simulink model "Test_model"  (R2022a)
settings: Solver=FixedStepAuto  StartTime=0.0  StopTime=.01  FixedStep=1e-6  RelTol=1e-3
libraries: spsSeriesRLCBranchLib x3, spsVoltageMeasurementLib x2, spsControlledVoltageSourceLib x1, simulink x1, spspowerguiLib x1
settings Model: Creator=ducks  LastModifiedBy=ducks

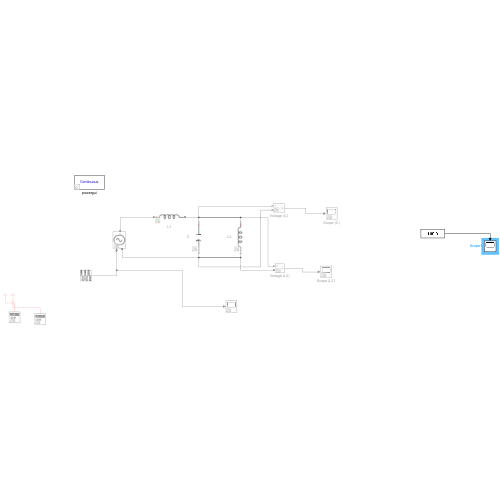
[thumbnail: Simulink's stored preview of the top-level diagram]
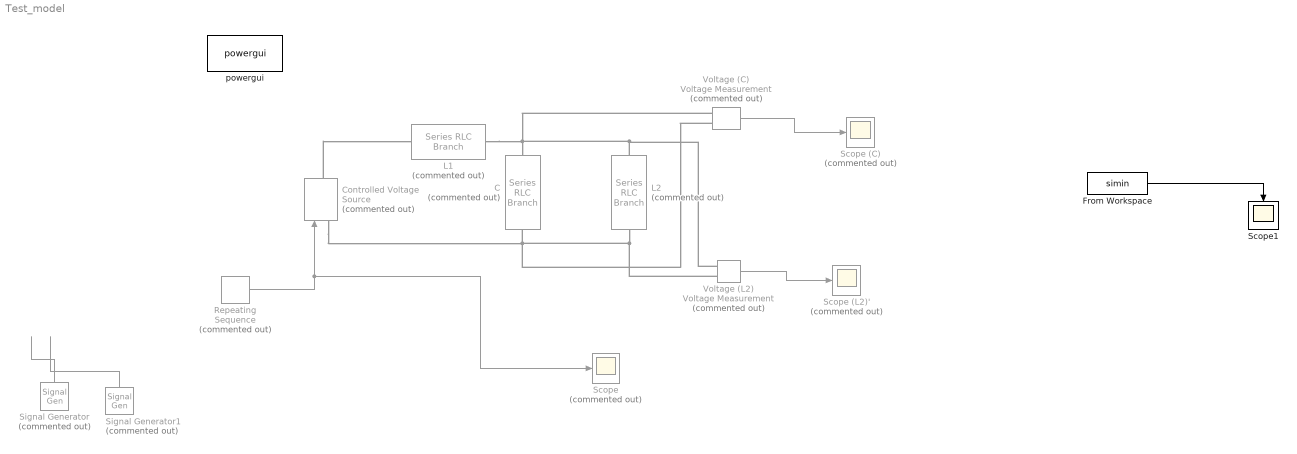
== system Test_model ==
  C : spsSeriesRLCBranchLib/Series RLC Branch  Commented=on  LConnTagsString=__new0  RConnTagsString=__new0  BranchType=C  Resistance=1  Inductance=1e-3  SetiL0=off  InitialCurrent=0  Capacitance=96e-6  Setx0=off  InitialVoltage=0  Measurements=None
  Controlled Voltage Source : spsControlledVoltageSourceLib/Controlled Voltage Source  Commented=on  Initialize=on  Source_Type=AC  Amplitude=0  Phase=0  Frequency=0  Measurements=None
  From Workspace : FromWorkspace  VariableName=simin
  L1 : spsSeriesRLCBranchLib/Series RLC Branch  Commented=on  LConnTagsString=__new0  RConnTagsString=__new0  BranchType=L  Resistance=1  Inductance=10e-6  SetiL0=off  InitialCurrent=0  Capacitance=0  Setx0=off  InitialVoltage=0  Measurements=None
  L2 : spsSeriesRLCBranchLib/Series RLC Branch  Commented=on  LConnTagsString=__new0  RConnTagsString=__new0  BranchType=L  Resistance=1  Inductance=2e-6  SetiL0=off  InitialCurrent=0  Capacitance=1e-6  Setx0=off  InitialVoltage=0  Measurements=None
  Repeating Sequence : simulink/Sources/Repeating Sequence  Commented=on  rep_seq_t=[0 .00002 .0000200001 .00004 .0000400001 .00006 .0000600001 .00009]  rep_seq_y=[0 0 1 1 0 0 -1 -1]
  Scope : Scope  Commented=on
  Scope (C) : Scope  Commented=on
  Scope (L2)' : Scope  Commented=on
  Scope1 : Scope
  Signal Generator : SignalGenerator  Commented=on  WaveForm=square  Units=rad/sec  VectorParams1D=off
  Signal Generator1 : SignalGenerator  Commented=on  WaveForm=square  Amplitude=-1  Units=rad/sec  VectorParams1D=off
  Voltage (C) : spsVoltageMeasurementLib/Voltage Measurement  Commented=on  PhasorSimulation=off  OutputType=Complex  PSBequivalent=0
  Voltage (L2) : spsVoltageMeasurementLib/Voltage Measurement  Commented=on  PhasorSimulation=off  OutputType=Complex  PSBequivalent=0
  powergui : spspowerguiLib/powergui  Priority=1  SimulationMode=Continuous  SampleTime=50e-6  frequency=60  Iterations=50  frequencyindice=0  Pbase=100e6  ErrMax=1e-4  UnitsV=kV  UnitsW=MW  buscounter=0  FunctionMessages=off  echomessages=off  EnableUseOfTLC=off  CurrentSourceSwitches=off  DisableSnubberDevices=off  DisableRonSwitches=off  DisableVfSwitches=off  DisplayEquations=off  AutomaticDiscreteSolvers=off  SolverType=Tustin/Backward Euler (TBE)  Interpol=off  ExternalGateDelay=off  methode=off  Ts=100  x0status=blocks  SPID=on  SwTol=0  HookPort=off  NonlinearTolerance=1e-4  nMaxIteration=100  ContinueOnMaxIteration=off  RestoreLinks=warning  ResistiveCurrentMeasurement=off  Frange=[0:2:500]  Ylog=off  Xlog=on  ShowGrid=off  save=off  variable=ZData  structure=0  ZoomFFT=off  StartTime=0.0  cycles=1  DisplayStyle=1  fundamental=60  FreqAxis=off  MaxFrequency=1000  frequencyindicesteady=1  RmsSteady=1  display=off
  wires:
  Voltage (C)/1 -> Scope (C)/1
  Voltage (L2)/1 -> Scope (L2)'/1
  Signal Generator/1 -> ?
  Signal Generator1/1 -> ?
  Repeating Sequence/1 -> Scope/1, Controlled Voltage Source/1
  From Workspace/1 -> Scope1/1
  connections:
  Controlled Voltage Source/RConn1 -- L1/LConn1
  Controlled Voltage Source/LConn1 -- Voltage (L2)/LConn2 -- L2/RConn1 -- Voltage (C)/LConn2 -- C/RConn1
  L1/RConn1 -- Voltage (L2)/LConn1 -- L2/LConn1 -- Voltage (C)/LConn1 -- C/LConn1
